simulink model "example_P_2"  (R2018a)
settings: Solver=VariableStepAuto  StartTime=0.0  StopTime=10.0  RelTol=1e-9
settings Model: Creator=gbecerra  LastModifiedBy=gbecerra

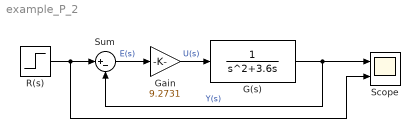
== system example_P_2 ==
  G(s) : TransferFcn  Denominator=[1 3.6 0]
  Gain : Gain  Gain=9.2731
  R(s) : Step  Time=0  SampleTime=0
  Scope : Scope  NumInputPorts=2
  Sum : Sum  Inputs=|+-
  wires:
  Sum/1 -> Gain/1  "E(s)"
  G(s)/1 -> Scope/1, Sum/2  "Y(s)"
  R(s)/1 -> Sum/1, Scope/2
  Gain/1 -> G(s)/1  "U(s)"
